simulink model "Project_simulation_revised"  (R2021a)
settings: Solver=VariableStepAuto  StartTime=0.0  StopTime=0.5  FixedStep=0.001  RelTol=1e-3  EnableMultiTasking=on
values from neighbouring files (symbols this model uses):
  a = l/(2*pi)/nthre/nthru    (= 0.00248679598581)    [Load_Parameter.m]
  d = 13600    [Load_Parameter.m]
  Jeq = m*l/(2*pi)+(JG+Jl)/a    (= 0.00653232609246)    [Load_Parameter.m]
  k = 40000    [Load_Parameter.m]
  l = 0.015    [Load_Parameter.m]
  Ld = 16e-3    (= 0.016)    [Load_Parameter.m]
  Lq = 16e-3    (= 0.016)    [Load_Parameter.m]
  Ls = 11.3e-3    (= 0.0113)    [Load_Parameter.m]
  PermanentMagnetFlux = 0.009    [Load_Parameter.m]
  Polepairs = 6    [Load_Parameter.m]
  RG = 32.23    [Load_Parameter.m]
  Th = 1/w_h    (= 0.00159154943092)    [Load_Parameter.m]
undefined symbols (not defined in the file or in its folder): sigbuilder_block
libraries: spsMosfetLib x6, spsVoltageMeasurementLib x3, spsDCVoltageSourceLib x2, spsNeutralLib x2, spsTriangleGeneratorLib x1, spspowerguiLib x1
settings Model: Creator=User  LastModifiedBy=61301765
settings SolverCC: SolverJacobianMethodControl=SparsePerturbation  AlgebraicLoopSolver=TrustRegion
settings DataIOCC: LimitDataPoints=on  SaveFormat=Array  ReturnWorkspaceOutputs=off
settings OptimizationCC: DefaultParameterBehavior=Inlined  EnhancedBackFolding=on  PassReuseOutputArgsAs=Individual arguments  OptimizeBlockOrder=speed  DifferentSizesBufferReuse=on  OptimizationCustomize=off  EfficientTunableParamExpr=on
settings DebuggingCC: UnderspecifiedInitializationDetection=Classic  MergeDetectMultiDrivingBlocksExec=none  SolverPrmCheckMsg=warning  ParameterTunabilityLossMsg=error  StateNameClashWarn=warning  SFUnexpectedBacktrackingDiag=warning  SFNoUnconditionalDefaultTransitionDiag=warning  SFExecutionAtInitializationDiag=none  SFMachineParentedDataDiag=warning  ArithmeticOperatorsInVariantConditions=warning
settings HardwareCC: ProdBitPerPointer=32  ProdBitPerSizeT=32  ProdBitPerPtrDiffT=32  ProdLargestAtomicFloat=None  ProdIntDivRoundTo=Undefined  ProdEndianess=Unspecified  ProdWordSize=32  ProdHWDeviceType=32-bit Generic
settings ModelReferenceCC: PropagateSignalLabelsOutOfModel=off
settings SFSimCC: SimUseLocalCustomCode=off  MATLABDynamicMemAlloc=off  CustomCodeUndefinedFunction=UseInterfaceOnly
settings RTWCC: SystemTargetFile=ert.tlc  TemplateMakefile=ert_default_tmf  GenerateReport=on  RTWUseLocalCustomCode=off  IncludeHyperlinkInReport=on  LaunchReport=on  GenerateTraceInfo=on  GenerateTraceReport=on  GenerateTraceReportSl=on  GenerateTraceReportSf=on  GenerateTraceReportEml=on
settings CodeAppCC: ForceParamTrailComments=on  IgnoreCustomStorageClasses=off  OperatorAnnotations=on  SimulinkDataObjDesc=on  SFDataObjDesc=on  InsertBlockDesc=on
settings ERTTargetCC: GenerateSampleERTMain=on  SupportContinuousTime=on  InlinedParameterPlacement=NonHierarchical  ERTCustomFileTemplate=example_file_process.tlc
settings ConfigComp: CovMetricSettings=dw  CovSaveCumulativeToWorkspaceVar=on  CovSaveSingleToWorkspaceVar=on  CovExternalEMLEnable=off

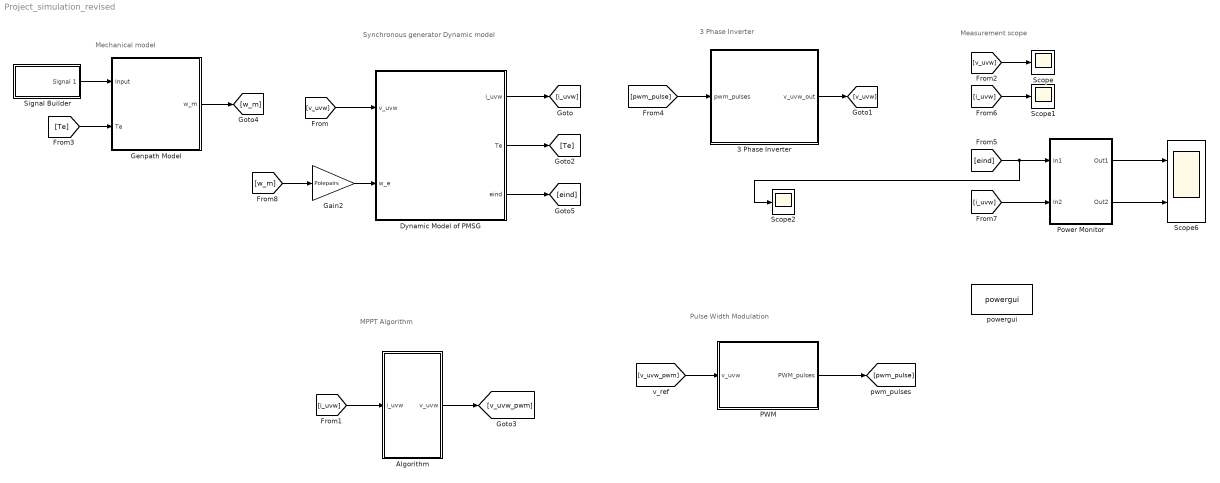
== system Project_simulation_revised ==
  note: Measurement scope
  note: 3 Phase Inverter
  note: Pulse Width Modulation
  note: Mechanical model
  note: Synchronous generator
      | Dynamic model
  note: MPPT Algorithm
  3 Phase Inverter : Subsystem
  Algorithm : Subsystem
  Dynamic Model of PMSG : Subsystem
  Gain2 : Gain  Gain=Polepairs
  Genpath Model : Subsystem
  PWM : Subsystem
  Power Monitor : Subsystem
  Scope : Scope
  Scope1 : Scope
  Scope2 : Scope
  Scope6 : Scope  NumInputPorts=2
  Signal Builder : Subsystem  Tag=STV Subsys  LoadFcn=sigbuilder_block('load',[1440 30 1440 722.25 ]);  StartFcn=sigbuilder_block('start');  StopFcn=sigbuilder_block('stop');  ClipboardFcn=sigbuilder_block('clipboard');  mask(Sigbuilder block){tuvar=[0:10]}
      mask help: Simulink:masks:SigbuilderBlock_MD
      mask init:
      | if ~strcmp(get_param(bdroot(gcbh),'SimulationStatus'),'stopped') tuvar = sigbuilder_block('maskInit'); end
      settings: CopyFcn=sigbuilder_block('copy');  DeleteFcn=sigbuilder_block('delete');  ModelCloseFcn=sigbuilder_block('modelClose');  PreSaveFcn=sigbuilder_block('preSave');  PauseFcn=sigbuilder_block('pause');  ContinueFcn=sigbuilder_block('continue');  NameChangeFcn=sigbuilder_block('namechange');  OpenFcn=sigbuilder_block('open',[6 30 1012.5 482.25 ]);  CloseFcn=sigbuilder_block('close');
      mask Display: plot(0, 0, 100, 100,[2, 2, 32, 32, 2], [68, 8, 8, 68, 68],[32, 2], [38, 38], [32, 19, 2],[53, 60, 44], [32, 17, 17, 2],[16, 16, 31, 31]);txt = getActiveGroup(gcbh);text(2, 100, txt,'verticalAlignment', 'top');
  powergui : spspowerguiLib/powergui  Priority=1  SimulationMode=Discrete  SampleTime=1e-6  frequency=60  Iterations=50  frequencyindice=0  Pbase=100e6  ErrMax=1e-4  UnitsV=kV  UnitsW=MW  buscounter=0  FunctionMessages=off  echomessages=off  EnableUseOfTLC=off  CurrentSourceSwitches=off  DisableSnubberDevices=off  DisableRonSwitches=off  DisableVfSwitches=off  DisplayEquations=off  AutomaticDiscreteSolvers=off  SolverType=Tustin/Backward Euler (TBE)  Interpol=off  ExternalGateDelay=off  methode=off  Ts=100  x0status=blocks  SPID=on  SwTol=0  HookPort=off  NonlinearTolerance=1e-4  nMaxIteration=100  ContinueOnMaxIteration=off  RestoreLinks=warning  ResistiveCurrentMeasurement=off  Frange=[0:2:500]  Ylog=off  Xlog=on  ShowGrid=off  save=off  variable=ZData  structure=voltagescope  ZoomFFT=off  StartTime=0.0  cycles=1  DisplayStyle=1  fundamental=100  FreqAxis=off  MaxFrequency=1500  frequencyindicesteady=1  RmsSteady=1  display=off
  wires:
  Dynamic Model of PMSG/2(Te) -> [Te]
  Gain2/1 -> Dynamic Model of PMSG/2(w_e)
  Dynamic Model of PMSG/1(i_uvw) -> [i_uvw]
  [v_uvw] -> Dynamic Model of PMSG/1(v_uvw)
  PWM/1(PWM_pulses) -> [pwm_pulse]
  [v_uvw_pwm] -> PWM/1(v_uvw)
  Algorithm/1(v_uvw) -> [v_uvw_pwm]
  [pwm_pulse] -> 3 Phase Inverter/1(pwm_pulses)
  3 Phase Inverter/1(v_uvw_out) -> [v_uvw]
  [i_uvw] -> Algorithm/1(i_uvw)
  [Te] -> Genpath Model/2(Te)
  Genpath Model/1(w_m) -> [w_m]
  [w_m] -> Gain2/1
  Dynamic Model of PMSG/3(eind) -> [eind]
  [eind] -> Scope2/1, Power Monitor/1(In1)
  [i_uvw] -> Power Monitor/2(In2)
  Power Monitor/1(Out1) -> Scope6/1
  Power Monitor/2(Out2) -> Scope6/2
  [v_uvw] -> Scope/1
  [i_uvw] -> Scope1/1
  Signal Builder/1(Signal 1) -> Genpath Model/1(Input)

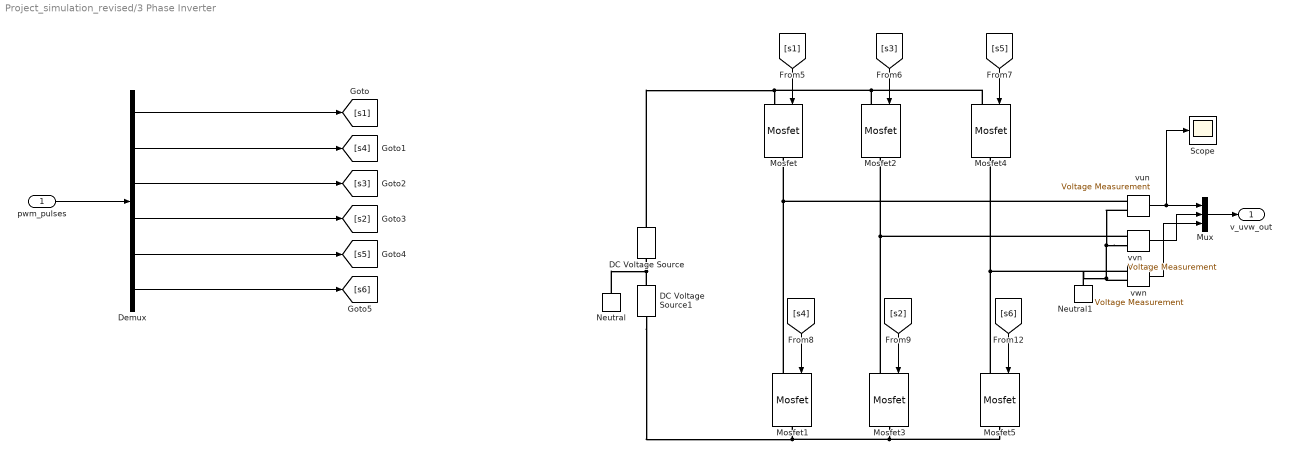
== system Project_simulation_revised/3 Phase Inverter ==
  pwm_pulses : Inport
  DC Voltage Source : spsDCVoltageSourceLib/DC Voltage Source  Amplitude=10  Measurements=None
  DC Voltage Source1 : spsDCVoltageSourceLib/DC Voltage Source  Amplitude=10  Measurements=None
  Demux : Demux  Outputs=6
  Mosfet{,1..5} (6 alike) : spsMosfetLib/Mosfet  Ron=0.1  Lon=0  Rd=0.01  Vfd=0  IC=0  Rs=1e5  Cs=inf  Measurements=off
  Mux : Mux  Inputs=3
  Neutral : spsNeutralLib/Neutral  LConnTagsString=a  NodeNumber=10
      settings: AttributesFormatString=node %<NodeNumber>  SourceProductBaseCode=PS
  Neutral1 : spsNeutralLib/Neutral  LConnTagsString=a  NodeNumber=10
      settings: AttributesFormatString=node %<NodeNumber>  SourceProductBaseCode=PS
  Scope : Scope
  vun : spsVoltageMeasurementLib/Voltage Measurement  PhasorSimulation=off  OutputType=Complex  PSBequivalent=0
  vvn : spsVoltageMeasurementLib/Voltage Measurement  PhasorSimulation=off  OutputType=Complex  PSBequivalent=0
  vwn : spsVoltageMeasurementLib/Voltage Measurement  PhasorSimulation=off  OutputType=Complex  PSBequivalent=0
  v_uvw_out : Outport
  wires:
  [s3] -> Mosfet2/1
  [s6] -> Mosfet5/1
  [s2] -> Mosfet3/1
  vwn/1 -> Mux/3
  Mux/1 -> v_uvw_out/1
  [s4] -> Mosfet1/1
  vun/1 -> Scope/1, Mux/1
  vvn/1 -> Mux/2
  [s1] -> Mosfet/1
  [s5] -> Mosfet4/1
  pwm_pulses/1 -> Demux/1
  Demux/1 -> [s1]
  Demux/2 -> [s4]
  Demux/3 -> [s3]
  Demux/4 -> [s2]
  Demux/5 -> [s5]
  Demux/6 -> [s6]
  connections:
  Mosfet1/LConn1 -- vun/LConn1 -- Mosfet/RConn1
  vvn/LConn2 -- vun/LConn2 -- Neutral1/LConn1 -- vwn/LConn2
  Mosfet3/LConn1 -- vvn/LConn1 -- Mosfet2/RConn1
  Mosfet/LConn1 -- DC Voltage Source/RConn1 -- Mosfet4/LConn1 -- Mosfet2/LConn1
  Mosfet3/RConn1 -- Mosfet5/RConn1 -- Mosfet1/RConn1 -- DC Voltage Source1/LConn1
  Mosfet5/LConn1 -- vwn/LConn1 -- Mosfet4/RConn1
  DC Voltage Source1/RConn1 -- Neutral/LConn1 -- DC Voltage Source/LConn1

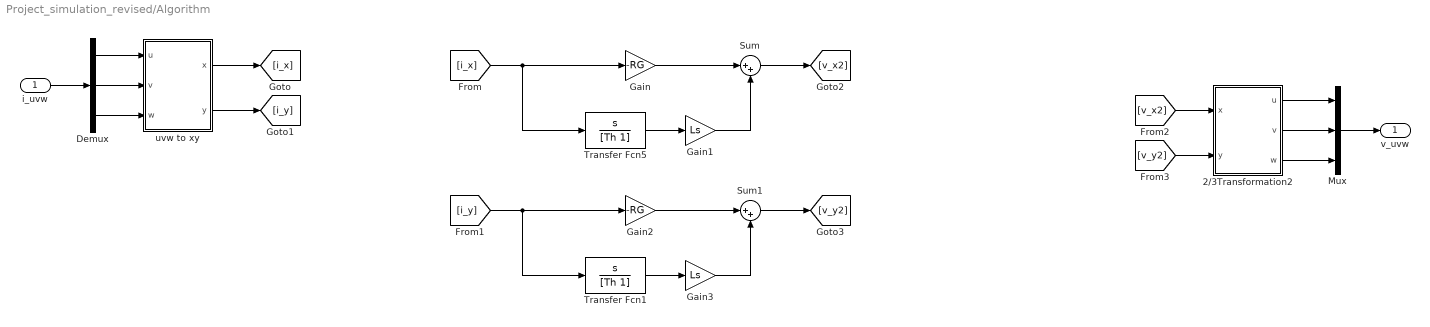
== system Project_simulation_revised/Algorithm ==
  i_uvw : Inport
  2/3Transformation2 : Subsystem
  Demux : Demux  Outputs=3
  Gain : Gain  Gain=-RG
  Gain1 : Gain  Gain=Ls
  Gain2 : Gain  Gain=-RG
  Gain3 : Gain  Gain=Ls
  Mux : Mux  Inputs=3
  Sum : Sum  Inputs=|++
  Sum1 : Sum  Inputs=|++
  Transfer Fcn1 : TransferFcn  Numerator=[1 0]  Denominator=[Th 1]
  Transfer Fcn5 : TransferFcn  Numerator=[1 0]  Denominator=[Th 1]
  uvw to xy : Subsystem
  v_uvw : Outport
  wires:
  i_uvw/1 -> Demux/1
  Demux/3 -> uvw to xy/3(w)
  Demux/2 -> uvw to xy/2(v)
  Demux/1 -> uvw to xy/1(u)
  uvw to xy/1(x) -> [i_x]
  uvw to xy/2(y) -> [i_y]
  [v_x2] -> 2/3Transformation2/1(x)
  [v_y2] -> 2/3Transformation2/2(y)
  2/3Transformation2/2(v) -> Mux/2
  2/3Transformation2/3(w) -> Mux/3
  2/3Transformation2/1(u) -> Mux/1
  Mux/1 -> v_uvw/1
  Gain/1 -> Sum/1
  [i_x] -> Transfer Fcn5/1, Gain/1
  Transfer Fcn5/1 -> Gain1/1
  Gain1/1 -> Sum/2
  Sum/1 -> [v_x2]
  Sum1/1 -> [v_y2]
  Gain3/1 -> Sum1/2
  Transfer Fcn1/1 -> Gain3/1
  [i_y] -> Gain2/1, Transfer Fcn1/1
  Gain2/1 -> Sum1/1

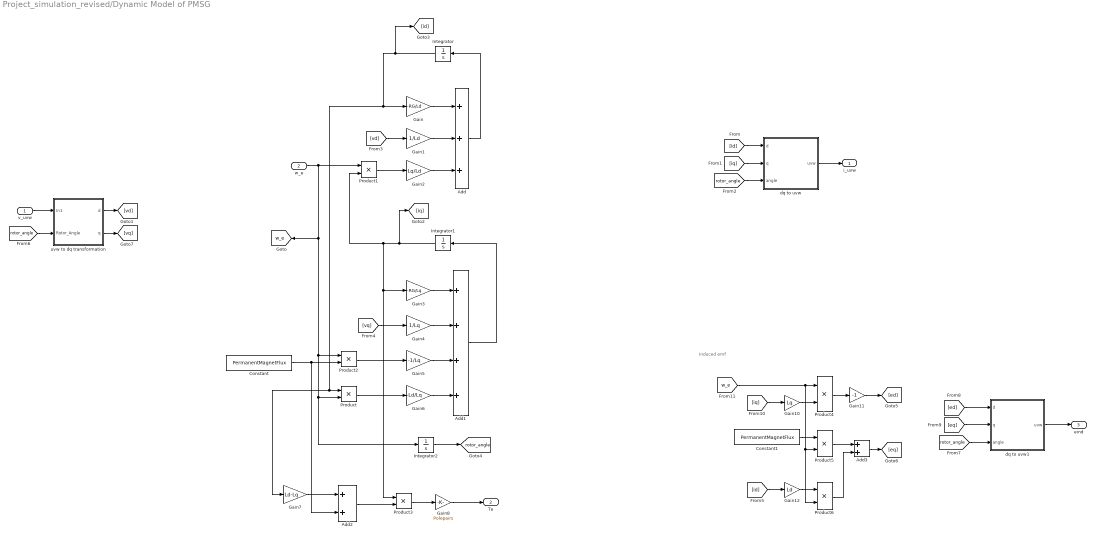
== system Project_simulation_revised/Dynamic Model of PMSG ==
  note: Induced emf
  v_uvw : Inport
  w_e : Inport  Port=2
  Add : Sum  Inputs=+++
  Add1 : Sum  Inputs=++++
  Add2 : Sum
  Add3 : Sum
  Constant : Constant  Value=PermanentMagnetFlux
  Constant1 : Constant  Value=PermanentMagnetFlux
  Gain : Gain  Gain=-RG/Ld
  Gain1 : Gain  Gain=1/Ld
  Gain10 : Gain  Gain=Lq
  Gain11 : Gain  Gain=-1
  Gain12 : Gain  Gain=Ld
  Gain2 : Gain  Gain=Lq/Ld
  Gain3 : Gain  Gain=-RG/Lq
  Gain4 : Gain  Gain=1/Lq
  Gain5 : Gain  Gain=-1/Lq
  Gain6 : Gain  Gain=-Ld/Lq
  Gain7 : Gain  Gain=Ld-Lq
  Gain8 : Gain  Gain=Polepairs
  Integrator : Integrator
  Integrator1 : Integrator
  Integrator2 : Integrator
  Product{,1..6} (7 alike) : Product
  dq to uvw : Subsystem
  dq to uvw1 : Subsystem
  uvw to dq transformation : Subsystem
  i_uvw : Outport
  Te : Outport  Port=2
  eind : Outport  Port=3
  tag scope: rotor_angle=global, w_e=global
  wires:
  Gain7/1 -> Add2/1
  Gain6/1 -> Add1/4
  Product1/1 -> Gain2/1
  [vq] -> Gain4/1
  Gain8/1 -> Te/1
  Product3/1 -> Gain8/1
  Product2/1 -> Gain5/1
  Gain1/1 -> Add/2
  Gain/1 -> Add/1
  Product/1 -> Gain6/1
  Gain5/1 -> Add1/3
  Gain2/1 -> Add/3
  Gain3/1 -> Add1/1
  Add2/1 -> Product3/2
  Add/1 -> Integrator/1
  Gain4/1 -> Add1/2
  Add1/1 -> Integrator1/1
  Integrator2/1 -> [rotor_angle]
  [id] -> dq to uvw/1(d)
  [iq] -> dq to uvw/2(q)
  [rotor_angle] -> dq to uvw/3(angle)
  dq to uvw/1(uvw) -> i_uvw/1
  [vd] -> Gain1/1
  Add3/1 -> [eq]
  Gain11/1 -> [ed]
  Integrator/1 -> [id], Gain/1, Gain7/1, Product/1
  Integrator1/1 -> [iq], Product1/2, Product3/1, Gain3/1
  Constant/1 -> Add2/2, Product2/2
  Gain10/1 -> Product4/2
  [ed] -> dq to uvw1/1(d)
  [rotor_angle] -> dq to uvw1/3(angle)
  [eq] -> dq to uvw1/2(q)
  w_e/1 -> Product/2, Integrator2/1, Product2/1, [w_e], Product1/1
  Product6/1 -> Add3/2
  Product4/1 -> Gain11/1
  dq to uvw1/1(uvw) -> eind/1
  Product5/1 -> Add3/1
  v_uvw/1 -> uvw to dq transformation/1(In1)
  [rotor_angle] -> uvw to dq transformation/2(Rotor_Angle)
  uvw to dq transformation/1(d) -> [vd]
  uvw to dq transformation/2(q) -> [vq]
  [id] -> Gain12/1
  [iq] -> Gain10/1
  [w_e] -> Product6/2, Product5/2, Product4/1
  Constant1/1 -> Product5/1
  Gain12/1 -> Product6/1

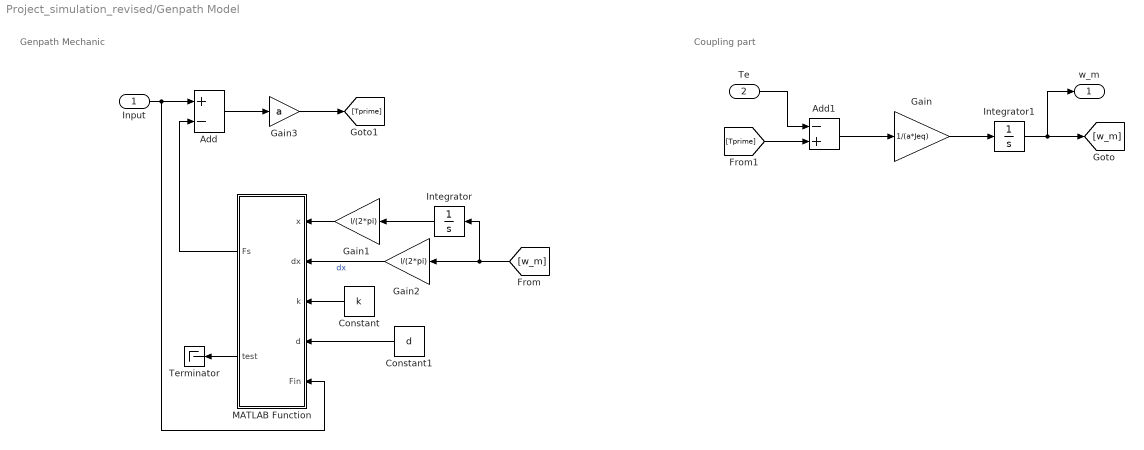
== system Project_simulation_revised/Genpath Model ==
  note: Coupling part
  note: Genpath Mechanic
  Input : Inport
  Te : Inport  Port=2
  Add : Sum  Inputs=+-
  Add1 : Sum  Inputs=-+
  Constant : Constant  Value=k
  Constant1 : Constant  Value=d
  Gain : Gain  Gain=1/(a*Jeq)
  Gain1 : Gain  Gain=l/(2*pi)
  Gain2 : Gain  Gain=l/(2*pi)
  Gain3 : Gain  Gain=a
  Integrator : Integrator
  Integrator1 : Integrator
  MATLAB Function : MATLAB Function  TreatAsAtomicUnit=on
  Terminator : Terminator
  w_m : Outport
  wires:
  Constant/1 -> MATLAB Function/3(k)
  Constant1/1 -> MATLAB Function/4(d)
  Gain2/1 -> MATLAB Function/2(dx)  "dx"
  Gain1/1 -> MATLAB Function/1(x)
  Gain3/1 -> [Tprime]
  Integrator/1 -> Gain1/1
  MATLAB Function/1(Fs) -> Add/2
  Input/1 -> MATLAB Function/5(Fin), Add/1
  Add/1 -> Gain3/1
  [w_m] -> Gain2/1, Integrator/1
  MATLAB Function/2(test) -> Terminator/1
  Te/1 -> Add1/1
  Add1/1 -> Gain/1
  Integrator1/1 -> w_m/1, [w_m]
  Gain/1 -> Integrator1/1
  [Tprime] -> Add1/2

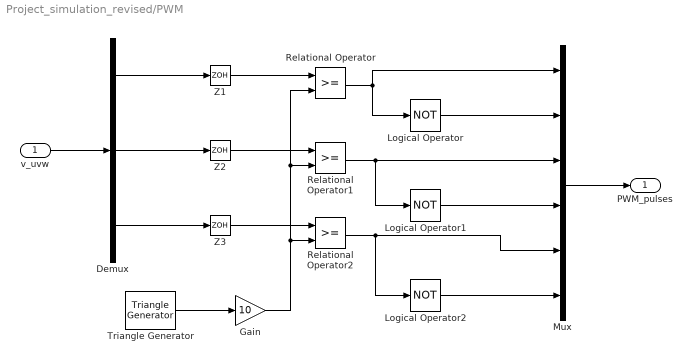
== system Project_simulation_revised/PWM ==
  v_uvw : Inport
  Demux : Demux  Outputs=3
  Gain : Gain  Gain=10
  Logical Operator : Logic  Operator=NOT  AllPortsSameDT=off  OutDataTypeStr=boolean
  Logical Operator1 : Logic  Operator=NOT  AllPortsSameDT=off  OutDataTypeStr=boolean
  Logical Operator2 : Logic  Operator=NOT  AllPortsSameDT=off  OutDataTypeStr=boolean
  Mux : Mux  Inputs=6
  Relational Operator : RelationalOperator  OutDataTypeStr=boolean  RndMeth=Simplest
  Relational Operator1 : RelationalOperator  OutDataTypeStr=boolean  RndMeth=Simplest
  Relational Operator2 : RelationalOperator  OutDataTypeStr=boolean  RndMeth=Simplest
  Triangle Generator : spsTriangleGeneratorLib/Triangle Generator  Freq=2e4  Phase=0  Ts=0
  Z1 : ZeroOrderHold  SampleTime=1/(2e4)
  Z2 : ZeroOrderHold  SampleTime=1/(2e4)
  Z3 : ZeroOrderHold  SampleTime=1/(2e4)
  PWM_pulses : Outport
  wires:
  Demux/3 -> Z3/1
  Z3/1 -> Relational Operator2/1
  Relational Operator2/1 -> Mux/5, Logical Operator2/1
  Demux/1 -> Z1/1
  Triangle Generator/1 -> Gain/1
  Z2/1 -> Relational Operator1/1
  Demux/2 -> Z2/1
  Gain/1 -> Relational Operator2/2, Relational Operator1/2, Relational Operator/2
  Relational Operator/1 -> Mux/1, Logical Operator/1
  Logical Operator1/1 -> Mux/4
  Logical Operator/1 -> Mux/2
  v_uvw/1 -> Demux/1
  Relational Operator1/1 -> Mux/3, Logical Operator1/1
  Logical Operator2/1 -> Mux/6
  Z1/1 -> Relational Operator/1
  Mux/1 -> PWM_pulses/1

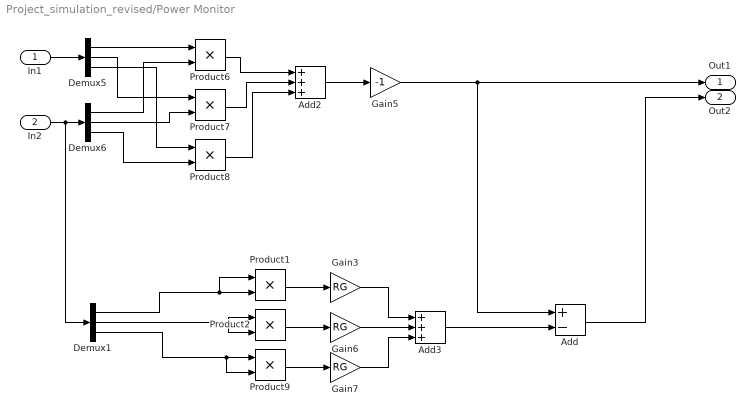
== system Project_simulation_revised/Power Monitor ==
  In1 : Inport
  In2 : Inport  Port=2
  Add : Sum  Inputs=+-
  Add2 : Sum  Inputs=+++
  Add3 : Sum  Inputs=+++
  Demux1 : Demux  Outputs=3
  Demux5 : Demux  Outputs=3
  Demux6 : Demux  Outputs=3
  Gain3 : Gain  Gain=RG
  Gain5 : Gain  Gain=-1
  Gain6 : Gain  Gain=RG
  Gain7 : Gain  Gain=RG
  Product{1..2,6..9} (6 alike) : Product
  Out1 : Outport
  Out2 : Outport  Port=2
  wires:
  Demux1/2 -> Product2/1, Product2/2
  Demux5/1 -> Product6/1
  Add2/1 -> Gain5/1
  In1/1 -> Demux5/1
  In2/1 -> Demux1/1, Demux6/1
  Demux1/3 -> Product9/2, Product9/1
  Product1/1 -> Gain3/1
  Product8/1 -> Add2/3
  Gain5/1 -> Out1/1, Add/1
  Demux6/1 -> Product6/2
  Demux1/1 -> Product1/1, Product1/2
  Product6/1 -> Add2/1
  Gain7/1 -> Add3/3
  Product7/1 -> Add2/2
  Product2/1 -> Gain6/1
  Demux6/3 -> Product8/2
  Gain3/1 -> Add3/1
  Add3/1 -> Add/2
  Gain6/1 -> Add3/2
  Product9/1 -> Gain7/1
  Demux5/3 -> Product8/1
  Demux5/2 -> Product7/1
  Demux6/2 -> Product7/2
  Add/1 -> Out2/1

== system Project_simulation_revised/Signal Builder ==
  Demux : Demux  Tag=STV Demux  Outputs=1
      settings: DisplayOption=none
  FromWs : FromWorkspace  Tag=STV FromWs  VariableName=tuvar
      SigBuilderData=|
      | common.afterFinalStr = 'Extrapolate'
      | common.sampleTime = 0
      | dataSet.timeRange = [0 10]
      | dataSet.name = 'Group 1'
      | sbobj.Groups.Name = 'Group 1'
      | sbobj.Groups.Signals.Name = 'Signal 1'
      | sbobj.Groups.Signals.XData = [0 0.025 0.05 0.15 0.25 10]
      | sbobj.Groups.Signals.YData = [0 810 965 920 0 10]
  Signal 1 : Outport  Tag=STV Outport  VectorParamsAs1DForOutWhenUnconnected=off
  wires:
  FromWs/1 -> Demux/1
  Demux/1 -> Signal 1/1

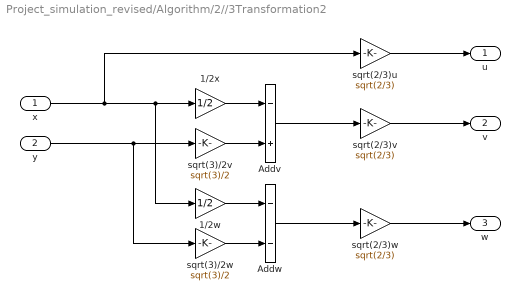
== system Project_simulation_revised/Algorithm/2//3Transformation2 ==
  x : Inport
  y : Inport  Port=2
  1/2w : Gain  Gain=1/2
  1/2x : Gain  Gain=1/2
  Addv : Sum  Inputs=-+
  Addw : Sum  Inputs=--
  sqrt(2/3)u : Gain  Gain=sqrt(2/3)
  sqrt(2/3)v : Gain  Gain=sqrt(2/3)
  sqrt(2/3)w : Gain  Gain=sqrt(2/3)
  sqrt(3)/2v : Gain  Gain=sqrt(3)/2
  sqrt(3)/2w : Gain  Gain=sqrt(3)/2
  u : Outport  VectorParamsAs1DForOutWhenUnconnected=off
  v : Outport  Port=2  VectorParamsAs1DForOutWhenUnconnected=off
  w : Outport  Port=3  VectorParamsAs1DForOutWhenUnconnected=off
  wires:
  x/1 -> sqrt(2/3)u/1, 1/2w/1, 1/2x/1
  sqrt(2/3)w/1 -> w/1
  sqrt(2/3)u/1 -> u/1
  1/2x/1 -> Addv/1
  y/1 -> sqrt(3)/2w/1, sqrt(3)/2v/1
  Addv/1 -> sqrt(2/3)v/1
  sqrt(3)/2w/1 -> Addw/2
  sqrt(3)/2v/1 -> Addv/2
  Addw/1 -> sqrt(2/3)w/1
  sqrt(2/3)v/1 -> v/1
  1/2w/1 -> Addw/1

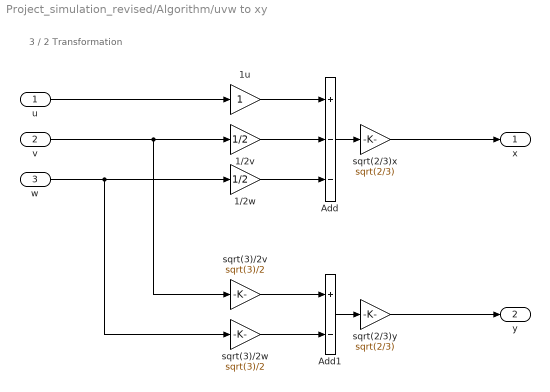
== system Project_simulation_revised/Algorithm/uvw to xy ==
  note: 3 / 2 Transformation
  u : Inport
  v : Inport  Port=2
  w : Inport  Port=3
  1/2v : Gain  Gain=1/2
  1/2w : Gain  Gain=1/2
  1u : Gain
  Add : Sum  Inputs=+--
  Add1 : Sum  Inputs=+-
  sqrt(2/3)x : Gain  Gain=sqrt(2/3)
  sqrt(2/3)y : Gain  Gain=sqrt(2/3)
  sqrt(3)/2v : Gain  Gain=sqrt(3)/2
  sqrt(3)/2w : Gain  Gain=sqrt(3)/2
  x : Outport  VectorParamsAs1DForOutWhenUnconnected=off
  y : Outport  Port=2  VectorParamsAs1DForOutWhenUnconnected=off
  wires:
  1/2v/1 -> Add/2
  1/2w/1 -> Add/3
  u/1 -> 1u/1
  w/1 -> sqrt(3)/2w/1, 1/2w/1
  v/1 -> sqrt(3)/2v/1, 1/2v/1
  1u/1 -> Add/1
  Add1/1 -> sqrt(2/3)y/1
  sqrt(3)/2v/1 -> Add1/1
  sqrt(2/3)x/1 -> x/1
  sqrt(3)/2w/1 -> Add1/2
  Add/1 -> sqrt(2/3)x/1
  sqrt(2/3)y/1 -> y/1

== system Project_simulation_revised/Dynamic Model of PMSG/dq to uvw ==
  d : Inport
  q : Inport  Port=2
  angle : Inport  Port=3
  2/3Transformation2 : Subsystem
  Mux2 : Mux  Inputs=3
  dq to xy2 : Subsystem
  uvw : Outport
  wires:
  2/3Transformation2/2(v) -> Mux2/2
  dq to xy2/2(y) -> 2/3Transformation2/2(y)
  d/1 -> dq to xy2/1(d)
  q/1 -> dq to xy2/2(q)
  2/3Transformation2/1(u) -> Mux2/1
  2/3Transformation2/3(w) -> Mux2/3
  angle/1 -> dq to xy2/3(Rotor_Angle)
  Mux2/1 -> uvw/1
  dq to xy2/1(x) -> 2/3Transformation2/1(x)

== system Project_simulation_revised/Dynamic Model of PMSG/dq to uvw1 ==
  d : Inport
  q : Inport  Port=2
  angle : Inport  Port=3
  2/3Transformation2 : Subsystem
  Mux2 : Mux  Inputs=3
  dq to xy2 : Subsystem
  uvw : Outport
  wires:
  2/3Transformation2/2(v) -> Mux2/2
  dq to xy2/2(y) -> 2/3Transformation2/2(y)
  d/1 -> dq to xy2/1(d)
  q/1 -> dq to xy2/2(q)
  2/3Transformation2/1(u) -> Mux2/1
  2/3Transformation2/3(w) -> Mux2/3
  angle/1 -> dq to xy2/3(Rotor_Angle)
  Mux2/1 -> uvw/1
  dq to xy2/1(x) -> 2/3Transformation2/1(x)

== system Project_simulation_revised/Dynamic Model of PMSG/uvw to dq transformation ==
  In1 : Inport
  Rotor_Angle : Inport  Port=2
  Demux1 : Demux  Outputs=3
  uvw to xy : Subsystem
  xy to dq : Subsystem
  d : Outport
  q : Outport  Port=2
  wires:
  Demux1/3 -> uvw to xy/3(w)
  Demux1/2 -> uvw to xy/2(v)
  uvw to xy/1(x) -> xy to dq/1(alpha)
  In1/1 -> Demux1/1
  uvw to xy/2(y) -> xy to dq/2(beta)
  Demux1/1 -> uvw to xy/1(u)
  xy to dq/2(q) -> q/1
  Rotor_Angle/1 -> xy to dq/3(Rotor_Angle)
  xy to dq/1(d) -> d/1

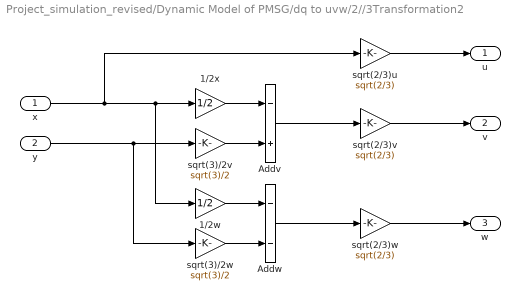
== system Project_simulation_revised/Dynamic Model of PMSG/dq to uvw/2//3Transformation2 ==
  x : Inport
  y : Inport  Port=2
  1/2w : Gain  Gain=1/2
  1/2x : Gain  Gain=1/2
  Addv : Sum  Inputs=-+
  Addw : Sum  Inputs=--
  sqrt(2/3)u : Gain  Gain=sqrt(2/3)
  sqrt(2/3)v : Gain  Gain=sqrt(2/3)
  sqrt(2/3)w : Gain  Gain=sqrt(2/3)
  sqrt(3)/2v : Gain  Gain=sqrt(3)/2
  sqrt(3)/2w : Gain  Gain=sqrt(3)/2
  u : Outport  VectorParamsAs1DForOutWhenUnconnected=off
  v : Outport  Port=2  VectorParamsAs1DForOutWhenUnconnected=off
  w : Outport  Port=3  VectorParamsAs1DForOutWhenUnconnected=off
  wires:
  x/1 -> sqrt(2/3)u/1, 1/2w/1, 1/2x/1
  sqrt(2/3)w/1 -> w/1
  sqrt(2/3)u/1 -> u/1
  1/2x/1 -> Addv/1
  y/1 -> sqrt(3)/2w/1, sqrt(3)/2v/1
  Addv/1 -> sqrt(2/3)v/1
  sqrt(3)/2w/1 -> Addw/2
  sqrt(3)/2v/1 -> Addv/2
  Addw/1 -> sqrt(2/3)w/1
  sqrt(2/3)v/1 -> v/1
  1/2w/1 -> Addw/1

== system Project_simulation_revised/Dynamic Model of PMSG/dq to uvw/dq to xy2 ==
  note: Axis transformation using flux phase angle
  d : Inport
  q : Inport  Port=2
  Rotor_Angle : Inport  Port=3
  Product{,1..3} (4 alike) : Product  InputSameDT=on  SaturateOnIntegerOverflow=on  OutDataTypeStr=Inherit: Same as first input
  Sum : Sum  Inputs=+-  InputSameDT=on  SaturateOnIntegerOverflow=on  OutDataTypeStr=Inherit: Same as first input
  Sum1 : Sum  InputSameDT=on  SaturateOnIntegerOverflow=on  OutDataTypeStr=Inherit: Same as first input
  cos : Fcn  Expr=cos(u)
  sine : Fcn  Expr=sin(u)
  x : Outport  VectorParamsAs1DForOutWhenUnconnected=off
  y : Outport  Port=2  VectorParamsAs1DForOutWhenUnconnected=off
  wires:
  cos/1 -> Product/2, Product2/2
  sine/1 -> Product1/2, Product3/2
  d/1 -> Product/1, Product3/1
  q/1 -> Product1/1, Product2/1
  Product1/1 -> Sum/2
  Product2/1 -> Sum1/1
  Product3/1 -> Sum1/2
  Product/1 -> Sum/1
  Sum/1 -> x/1
  Sum1/1 -> y/1
  Rotor_Angle/1 -> cos/1, sine/1

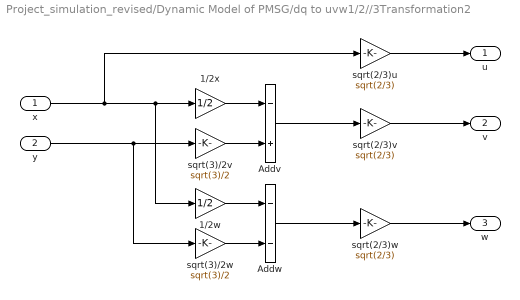
== system Project_simulation_revised/Dynamic Model of PMSG/dq to uvw1/2//3Transformation2 ==
  x : Inport
  y : Inport  Port=2
  1/2w : Gain  Gain=1/2
  1/2x : Gain  Gain=1/2
  Addv : Sum  Inputs=-+
  Addw : Sum  Inputs=--
  sqrt(2/3)u : Gain  Gain=sqrt(2/3)
  sqrt(2/3)v : Gain  Gain=sqrt(2/3)
  sqrt(2/3)w : Gain  Gain=sqrt(2/3)
  sqrt(3)/2v : Gain  Gain=sqrt(3)/2
  sqrt(3)/2w : Gain  Gain=sqrt(3)/2
  u : Outport  VectorParamsAs1DForOutWhenUnconnected=off
  v : Outport  Port=2  VectorParamsAs1DForOutWhenUnconnected=off
  w : Outport  Port=3  VectorParamsAs1DForOutWhenUnconnected=off
  wires:
  x/1 -> sqrt(2/3)u/1, 1/2w/1, 1/2x/1
  sqrt(2/3)w/1 -> w/1
  sqrt(2/3)u/1 -> u/1
  1/2x/1 -> Addv/1
  y/1 -> sqrt(3)/2w/1, sqrt(3)/2v/1
  Addv/1 -> sqrt(2/3)v/1
  sqrt(3)/2w/1 -> Addw/2
  sqrt(3)/2v/1 -> Addv/2
  Addw/1 -> sqrt(2/3)w/1
  sqrt(2/3)v/1 -> v/1
  1/2w/1 -> Addw/1

== system Project_simulation_revised/Dynamic Model of PMSG/dq to uvw1/dq to xy2 ==
  note: Axis transformation using flux phase angle
  d : Inport
  q : Inport  Port=2
  Rotor_Angle : Inport  Port=3
  Product{,1..3} (4 alike) : Product  InputSameDT=on  SaturateOnIntegerOverflow=on  OutDataTypeStr=Inherit: Same as first input
  Sum : Sum  Inputs=+-  InputSameDT=on  SaturateOnIntegerOverflow=on  OutDataTypeStr=Inherit: Same as first input
  Sum1 : Sum  InputSameDT=on  SaturateOnIntegerOverflow=on  OutDataTypeStr=Inherit: Same as first input
  cos : Fcn  Expr=cos(u)
  sine : Fcn  Expr=sin(u)
  x : Outport  VectorParamsAs1DForOutWhenUnconnected=off
  y : Outport  Port=2  VectorParamsAs1DForOutWhenUnconnected=off
  wires:
  cos/1 -> Product/2, Product2/2
  sine/1 -> Product1/2, Product3/2
  d/1 -> Product/1, Product3/1
  q/1 -> Product1/1, Product2/1
  Product1/1 -> Sum/2
  Product2/1 -> Sum1/1
  Product3/1 -> Sum1/2
  Product/1 -> Sum/1
  Sum/1 -> x/1
  Sum1/1 -> y/1
  Rotor_Angle/1 -> cos/1, sine/1

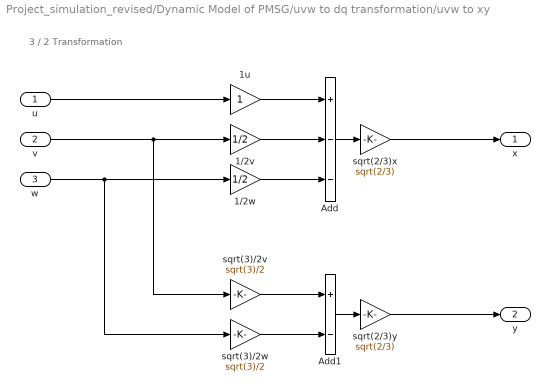
== system Project_simulation_revised/Dynamic Model of PMSG/uvw to dq transformation/uvw to xy ==
  note: 3 / 2 Transformation
  u : Inport
  v : Inport  Port=2
  w : Inport  Port=3
  1/2v : Gain  Gain=1/2
  1/2w : Gain  Gain=1/2
  1u : Gain
  Add : Sum  Inputs=+--
  Add1 : Sum  Inputs=+-
  sqrt(2/3)x : Gain  Gain=sqrt(2/3)
  sqrt(2/3)y : Gain  Gain=sqrt(2/3)
  sqrt(3)/2v : Gain  Gain=sqrt(3)/2
  sqrt(3)/2w : Gain  Gain=sqrt(3)/2
  x : Outport  VectorParamsAs1DForOutWhenUnconnected=off
  y : Outport  Port=2  VectorParamsAs1DForOutWhenUnconnected=off
  wires:
  1/2v/1 -> Add/2
  1/2w/1 -> Add/3
  u/1 -> 1u/1
  w/1 -> sqrt(3)/2w/1, 1/2w/1
  v/1 -> sqrt(3)/2v/1, 1/2v/1
  1u/1 -> Add/1
  Add1/1 -> sqrt(2/3)y/1
  sqrt(3)/2v/1 -> Add1/1
  sqrt(2/3)x/1 -> x/1
  sqrt(3)/2w/1 -> Add1/2
  Add/1 -> sqrt(2/3)x/1
  sqrt(2/3)y/1 -> y/1

== system Project_simulation_revised/Dynamic Model of PMSG/uvw to dq transformation/xy to dq ==
  note: Inverse axis transformation
      | using flux phase angle
  alpha : Inport
  beta : Inport  Port=2
  Rotor_Angle : Inport  Port=3
  Product{,1..3} (4 alike) : Product  InputSameDT=on  SaturateOnIntegerOverflow=on  OutDataTypeStr=Inherit: Same as first input
  Sum : Sum  Inputs=+-  InputSameDT=on  SaturateOnIntegerOverflow=on  OutDataTypeStr=Inherit: Same as first input
  Sum1 : Sum  InputSameDT=on  SaturateOnIntegerOverflow=on  OutDataTypeStr=Inherit: Same as first input
  cos : Fcn  Expr=cos(-u)
  sine : Fcn  Expr=sin(-u)
  d : Outport  VectorParamsAs1DForOutWhenUnconnected=off
  q : Outport  Port=2  VectorParamsAs1DForOutWhenUnconnected=off
  wires:
  cos/1 -> Product/2, Product2/2
  sine/1 -> Product1/2, Product3/2
  alpha/1 -> Product/1, Product3/1
  beta/1 -> Product1/1, Product2/1
  Product1/1 -> Sum/2
  Product2/1 -> Sum1/1
  Product3/1 -> Sum1/2
  Product/1 -> Sum/1
  Rotor_Angle/1 -> cos/1, sine/1
  Sum/1 -> d/1
  Sum1/1 -> q/1

== matlab function Project_simulation_revised/Genpath Model/MATLAB Function ==
  data: x input; dx input; k input; d input; Fs output; Fin input; test output
function [Fs,test] = fcn(x,dx,k,d,Fin)

if x >-0.015
    Fs = k*x+d*dx;
    test = 1;
else
    Fs = Fin+d*dx;
    test = 0;
end
if Fin == 0
    Fs = k*x+d*dx;
    test = 2;
end
